simulink model "test_Simulink"  (R2019b)
settings: Solver=VariableStepAuto  StartTime=0.0  StopTime=10.0  RelTol=1e-3
values from neighbouring files (symbols this model uses):
  Amp = 10    [test_Simulink.m]
  f = f1*i    [sim_LIM.m]    (also in test_Simulink.m = 0.1)
settings Model: Creator=max_m  LastModifiedBy=max_m

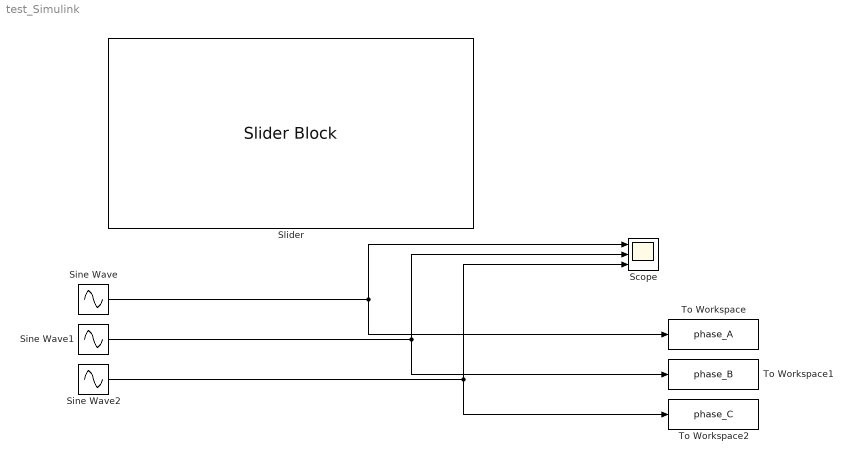
== system test_Simulink ==
  Scope : Scope  NumInputPorts=3
  Sine Wave : Sin  Amplitude=Amp  Frequency=2*pi*f  SampleTime=0
  Sine Wave1 : Sin  Amplitude=Amp  Frequency=2*pi*f  Phase=2*pi/3  SampleTime=0
  Sine Wave2 : Sin  Amplitude=Amp  Frequency=2*pi*f  Phase=-2*pi/3  SampleTime=0
  Slider : SliderBlock
  To Workspace : ToWorkspace  VariableName=phase_A  SaveFormat=Timeseries  SampleTime=-1
  To Workspace1 : ToWorkspace  VariableName=phase_B  SaveFormat=Timeseries  SampleTime=-1
  To Workspace2 : ToWorkspace  VariableName=phase_C  SaveFormat=Timeseries  SampleTime=-1
  wires:
  Sine Wave/1 -> To Workspace/1, Scope/1
  Sine Wave1/1 -> Scope/2, To Workspace1/1
  Sine Wave2/1 -> Scope/3, To Workspace2/1
